simulink model "SF015A_WhlImbRejctn"  (R2013b)
settings: Solver=FixedStepDiscrete  SolverMode=SingleTasking  StartTime=0.0  StopTime=1  FixedStep=0.002  RelTol=1e-3
undefined symbols (not defined in the file): ACTIVBANDMAX_ULS_U32, ADAPVFILMAX_ULS_F32, ADJOUTPMAX_ULS_F32, ARCHGLBPRM_180OVERPI_ULS_F32, ARCHGLBPRM_2MILLISEC_SEC_F32, ARCHGLBPRM_2PI_ULS_F32, ARCHGLBPRM_FLOATZEROTHD_ULS_F32, ARCHGLBPRM_PI_ULS_F32, ARCHGLBPRM_PIOVER180_ULS_F32, ARCHGLBPRM_PIOVER2_ULS_F32, CALMINSPERCOUNT_ULS_F32, Cntr, DURATIONDISABLE_CNT_U16, FILTWHLSPDMAX_MOTRADPERSEC_F32, FRQMIN_ULS_F32, MICROSECTOMILLISEC_ULS_F32, MINSTOMILLISEC_ULS_F32, NINETY_ULS_F32, NODEBSTEP_CNT_U16, NROFDLY_CNT_U08, NtcSts1, NvmGetErrSts1, ONEHALF_ULS_F32, ONEHUNDRED_ULS_F32, ONEOVRTHREE_ULS_F32, ONEOVRTWENTY_ULS_F32, ONETHOUSAND_ULS_F32, PEAKMAX_ULS_F32, PEAKMIN_ULS_F32, PHAADJMAX_ULS_F32, PITIMESSAMPLETIME_ULS_F32, SigQlfr1, STOREDMINSPERCOUNT_ULS_F32, Sts, SysSt1, TWO_ULS_F32, TWOOVRTHREE_ULS_F32, UGRFILMAX_ULS_F32, WhlImbRejctnAdpvFac, WhlImbRejctnAutScaEna, WhlImbRejctnAutScaTar, WhlImbRejctnCurrMgnSlewPerLoop, WhlImbRejctnDcTrendFltRcvryDly, WhlImbRejctnDcTrendFltRcvryNegStep, WhlImbRejctnDcTrendFltRcvryPosStep, WhlImbRejctnDcTrendFltRcvryThd, WhlImbRejctnDcTrendTh2Tq, WhlImbRejctnDcTrendThTq, WhlImbRejctnDcTrendTi2Sec, WhlImbRejctnDcTrendTiSec, WhlImbRejctnEnaSlewPerLoop, WhlImbRejctnFctEna, WhlImbRejctnFltNtc, WhlImbRejctnFrqDiagcAmpThd, WhlImbRejctnFrqDiagcEna, WhlImbRejctnFrqDiagcFltRcvryDly, WhlImbRejctnFrqDiagcFltRcvryNegStep, WhlImbRejctnFrqDiagcFltRcvryPosStep, WhlImbRejctnFrqDiagcFltRcvryThd, WhlImbRejctnFrqDiagcThd ... (+30)
libraries: FixdToFloat x32, simulink x26, NxtrLim x25, Fil x20, NxtrAbslt x9, NxtrMath x7, NxtrMax x6, NxtrMin x4, NxtrNvM x2, FloatToFixd x2, LnrIntrpn x2, NxtrSign x1
(part 1 of 14)
settings Model: Creator=VZBTJX  LastModifiedBy=XZB1DB
settings SolverCC: AutoInsertRateTranBlk=on  InsertRTBMode=Always
settings DataIOCC: LimitDataPoints=off  SaveFormat=Structure  ReturnWorkspaceOutputs=on
settings OptimizationCC: BlockReduction=off  InlineParams=on  ZeroExternalMemoryAtStartup=off  ZeroInternalMemoryAtStartup=off  OptimizeModelRefInitCode=on  LifeSpan=1
settings DebuggingCC: SignalInfNanChecking=error  SignalRangeChecking=warning  UnderspecifiedInitializationDetection=Simplified  SolverPrmCheckMsg=error  InheritedTsInSrcMsg=error  DiscreteInheritContinuousMsg=error  SingleTaskRateTransMsg=error  TasksWithSamePriorityMsg=error  SigSpecEnsureSampleTimeMsg=error  CheckMatrixSingularityMsg=error  ParameterUnderflowMsg=error  ParameterPrecisionLossMsg=error  ParameterTunabilityLossMsg=error  FixptConstUnderflowMsg=warning  FixptConstOverflowMsg=warning  VectorMatrixConversionMsg=error  SignalLabelMismatchMsg=error  UnconnectedInputMsg=error  UnconnectedOutputMsg=error  UnconnectedLineMsg=error  SFcnCompatibilityMsg=error  UniqueDataStoreMsg=warning  BusObjectLabelMismatch=error  RootOutportRequireBusObject=error  AssertControl=DisableAll  ModelReferenceIOMsg=error  ModelReferenceVersionMismatchMessage=warning  ModelReferenceIOMismatchMessage=error  ModelReferenceCSMismatchMessage=warning  ModelReferenceDataLoggingMessage=error  StateNameClashWarn=warning  StrictBusMsg=ErrorOnBusTreatedAsVector  NonBusSignalsTreatedAsBus=error  SFUnexpectedBacktrackingDiag=error  SFInvalidInputDataAccessInChartInitDiag=error  SFNoUnconditionalDefaultTransitionDiag=error  SFTransitionOutsideNaturalParentDiag=error  SFUnconditionalTransitionShadowingDiag=error  SFUndirectedBroadcastEventsDiag=error
settings ModelReferenceCC: ModelReferenceNumInstancesAllowed=Single
settings RTWCC: SystemTargetFile=autosar.tlc  GenCodeOnly=on  TemplateMakefile=ert_default_tmf  Description=AUTOSAR  GenerateReport=on  ProcessScript=autosar_make_rtw_hook  LaunchReport=on
settings CodeAppCC: GenerateComments=off  IgnoreCustomStorageClasses=off  CustomSymbolStrType=$N$R$M  CustomSymbolStrBlkIO=$N$M  SimulinkBlockComments=off
settings STFCustomTargetCC: ParMdlRefBuildCompliant=on  CompOptLevelCompliant=on  IncludeMdlTerminateFcn=off  CombineOutputUpdateFcns=on  SuppressErrorStatus=on  ERTFirstTimeCompliant=on  ERTCustomFileBanners=on  SupportNonFinite=off  SupportComplex=off  SupportContinuousTime=off  SupportNonInlinedSFcns=off  MATLABClassNameForMDSCustomization=Simulink.SoftwareTarget.ERTCustomization  AutosarCompliant=on  GRTInterface=off  SystemTargetFile=autosar.tlc
settings ERTTargetCC: CodeReplacementLibrary=ANSI_C  ConcurrentExecutionCompliant=off  IncludeMdlTerminateFcn=off  SuppressErrorStatus=on  SupportNonFinite=off  SupportComplex=off  ModelStepFunctionPrototypeControlCompliant=off  CPPClassGenCompliant=off  AutosarCompliant=on  InlinedParameterPlacement=NonHierarchical  ERTCustomFileTemplate=example_file_process.tlc  EnableUserReplacementTypes=on

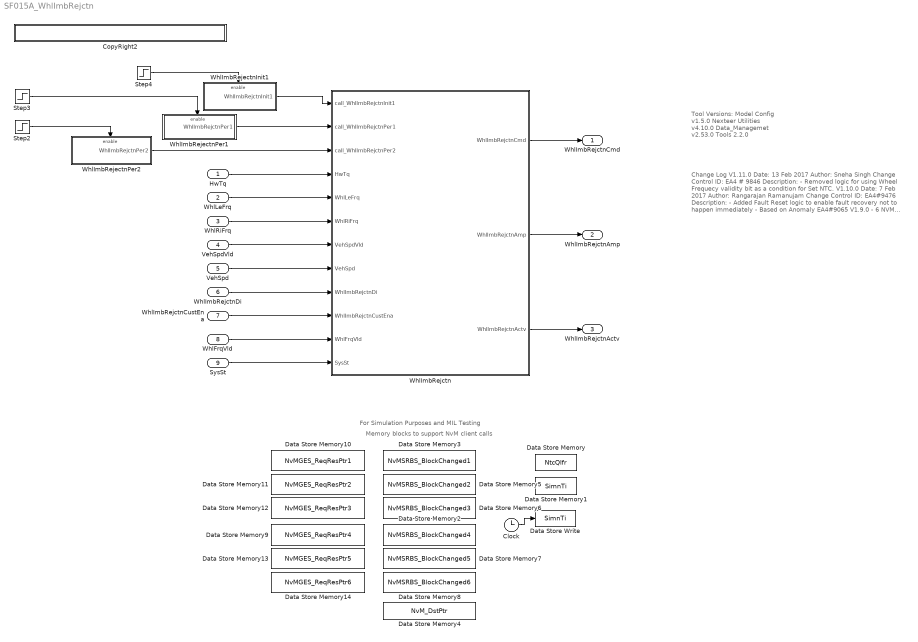
== system SF015A_WhlImbRejctn ==
  note: Tool Versions:
      |
      | Model Config v1.5.0
      | Nexteer Utilities v4.10.0
      | Data_Managemet v2.53.0
      | Tools 2.2.0
  note: Change Log
      |
      | V1.11.0
      | Date: 13 Feb 2017
      | Author: Sneha Singh
      | Change Control ID: EA4 # 9846
      | Description:
      | - Removed logic for using Wheel Frequecy validity bit as a condition for Set NTC.
      |
      | V1.10.0
      | Date: 7 Feb 2017
      | Author: Rangarajan Ramanujam
      | Change Control ID: EA4#9476
      | Description:
      | - Added Fault Reset logic to enable fault recovery not to happen immediately
      | - Based on Anomaly EA4#9065
      |
      |
      | V1.9.0
      | - 6 NVM variables corresponding to Struct 1 NVM block(CmpPeakData).
      | - FRQMIN_ULS_F32 constant added in DD and Model
      | - Input and Output Ports promoted at the top level per Std.
      | - Precision updated  for WhlFreq InRange and WhlFreq InRange 1 Subsystem
      |
      |
      | V1.8.0
      | Date: 28 Nov 2016
      | Author: Rangarajan Ramanujam
      | Change Control ID: EA4#8201
      | Description:
      | - EngMax of DlyIdxLe and DlyIdxRi updated in DD.
      | - Updated the range of PIMs in DD.
      | - Updated IRV properties in DD for 'IniCmpFlt'.
      | - Modified the  '<=' to '>' in PeakLe and PeakRi blocks. The problem exists
      | only in model. No change to code
      | - Updated the EngVal of 'DURATIONDISABLE_CNT_U16' in DD.
      | - Tapped delay implementation has been modified.
      | - Phase Adjust block has been modified.
      | - Updated the block 'Active Rejection Command'.
      | - Modified the Adaptive Filter blocks.
      | - Updated the UGR filter logic.
      | - Deleted few PIMs
      | - Reset WIR block has been updated.
      | - Updated Set NTC blocks without trigger from latest tools
      | - Changed constant value of 'MICROSECTOMILLISEC_ULS_F32' from 0.001 to 0.1
      |
      |
      |
      | V1.7.0
      | Date: 11 October 2016
      | Author: Rangarajan Ramanujam
      | Change Control ID: EA4#7923
      | Description:
      | - PIM Ranges in 'Slow Speed Diagc' update in Data dictionary
      | - Logic update in Data dictionary for not updating PIM when value is at
      | data type max
      | - Add Compensation fault diagnostic to init as per EA3 code
      | - Change NVM checking condition in Init to data type max of u32 instead of
      | u16
      | -The Lowpass filter variable for computing CurrMagLe and CurrMagRi
      | were same and this was resolved with separate Low pass filter state
      | variables for Le and Ri.
      | - Logic for Enabling and disabling WIR updated/changed as per Ea3 code
      |
      | V1.6.0
      | - Minimum Value of LpFil variables checked and changed to prevent
      |  divide by zero issues
      | - Latest tools used to fix LpFil error and prevent LpFilGain being
      | set to zero
      | - Display variable write blocks missing were updated :
      | dWhlImbRejctnLMSqdOutLe and dWhlImbRejctnLMSqdOutRi
      | - Pim Data store memory blocks Diagnostics set to 'none'
      | - Width block used to select first and last elements of an array
      | instead of using 'Arrayname(1)' or 'Arrayname(end)'
      |
      | V1.5.0
      | - 'OR' block replaced with 'Bitwise OR' in the subsystem 'WIR
      | Diagnostics/Set NTC Block'.
      | - Updated the datatype of NTC failure bits to 'uint8' in the 'WIR
      | Diagnostics/Set NTC Block'.
      | - Logic for setting of NTC bit based on WheelFrequencyValid
      | signal has been removed from the subsystem 'WIR Diagnostics'.
      | - Properties of few simulink blocks have been changed to make
      | the model simulatable.
      | - The definition of PIMs of type'Bus:PassFailCntrDiagcRec1' has
      | been updated in the data dictionary.
      |
      |
      | V1.4.0
      | Date: 01 August 2016
      | Author: Rangarajan Ramanujam
      | Change Control: 6681
      | Description:
      | - Rearranging design logic in Wheel speed Correlation check
      |  to remove redundant checks and  match code with model
      |
      | v1.3.0
      | Date: 6 June 2016
      | Author: Sneha Singh
      | Change Control ID: EA4# 5952
      | - NOT block added to the signal WhlImbRejctnDi
      | - Elapsed timer comparison modified from '<=' to '>='.
      | - Changed units of few cals from 'Milliseconds' to 'Mins'.
      | - Logic for conversion of minutes to milliseconds added.
      | - Added a new constant for minutes to milliseconds conversion.
      |
      | V1.2.0
      | Date: 23 Mar 2016
      | Author :Rangarajan Ramanujam
      | Change control :
      | Description:
      | - NVM checks added
      | - Typos fixed in cal names
      | - Design changes in Phase adjust
      | - Initial values updated according to review
      |
      | V1.1.0
      | -Changes corresponding to software review
      |
      | V1.0.0
      | - Initial Release
      | - Based on EA3 Word doc
      | - Level 3 Model
  note: For Simulation Purposes and MIL Testing
  note: Memory blocks to support NvM client calls
  HwTq : Inport
  WhlLeFrq : Inport  Port=2
  WhlRiFrq : Inport  Port=3
  VehSpdVld : Inport  Port=4
  VehSpd : Inport  Port=5
  WhlImbRejctnDi : Inport  Port=6
  WhlImbRejctnCustEna : Inport  Port=7
  WhlFrqVld : Inport  Port=8
  SysSt : Inport  Port=9
  Clock : Clock
  CopyRight2 : Subsystem  Description=|  mask(Copyright Information){none=on}
      | Copyright info block.                                               
      |                                                                     
      | Place copyright information at the top of every subsystem in design.
      mask prompts: none "No parameters"
      mask help: Place copyright information at the top of every subsystem in design.
      mask Display:
      | NxtrConf = 'Nexteer Confidential';
      | 
      | sys = bdroot; %handle for the current model ("system")
      | first = get_param(sys,'Created');
      | first = first(end-3:end);  %year is last four digits
      | 
      | last = get_param(sys,'LastModifiedDate');
      | if isempty(last)
      |     last = datestr(now,'yyyy');
      | else
      |     last = last(end-3:end);
      | end
      | 
      | if strcmp(first,last)
      |     fprintf('%s -- Copyright %s Nexteer',NxtrConf,first)
      | else
      |     fprintf('%s -- %s%s- %s Nexteer',NxtrConf,char(169),first,last)
      | end
  Data Store Memory : DataStoreMemory  DataStoreName=NtcQlfr
  Data Store Memory1 : DataStoreMemory  DataStoreName=SimnTi
  Data Store Memory10 : DataStoreMemory  DataStoreName=NvMGES_ReqResPtr1
  Data Store Memory11 : DataStoreMemory  DataStoreName=NvMGES_ReqResPtr2
  Data Store Memory12 : DataStoreMemory  DataStoreName=NvMGES_ReqResPtr3
  Data Store Memory13 : DataStoreMemory  DataStoreName=NvMGES_ReqResPtr5
  Data Store Memory14 : DataStoreMemory  DataStoreName=NvMGES_ReqResPtr6
  Data Store Memory2 : DataStoreMemory  DataStoreName=NvMSRBS_BlockChanged4
  Data Store Memory3 : DataStoreMemory  DataStoreName=NvMSRBS_BlockChanged1
  Data Store Memory4 : DataStoreMemory  DataStoreName=NvM_DstPtr
  Data Store Memory5 : DataStoreMemory  DataStoreName=NvMSRBS_BlockChanged2
  Data Store Memory6 : DataStoreMemory  DataStoreName=NvMSRBS_BlockChanged3
  Data Store Memory7 : DataStoreMemory  DataStoreName=NvMSRBS_BlockChanged5
  Data Store Memory8 : DataStoreMemory  DataStoreName=NvMSRBS_BlockChanged6
  Data Store Memory9 : DataStoreMemory  DataStoreName=NvMGES_ReqResPtr4
  Data Store Write : DataStoreWrite  DataStoreName=SimnTi
  Step2 : Step  Time=0  SampleTime=0.004
  Step3 : Step  Time=0  SampleTime=0.002
  Step4 : Step  Time=0  Before=1  After=0  SampleTime=0.002
  WhlImbRejctn : Subsystem
  WhlImbRejectnInit1 : Subsystem  RequirementInfo={} %GIDa_18617733_e4ee_4886_bcc3_385a7dcf992d  TreatAsAtomicUnit=on
  WhlImbRejectnPer1 : Subsystem  RequirementInfo={} %GIDa_501e26ae_c5a8_44f7_acd8_34ad9ece32fe  TreatAsAtomicUnit=on
  WhlImbRejectnPer2 : Subsystem  RequirementInfo={} %GIDa_04db69de_43d9_4850_9e5a_188d21d54238  TreatAsAtomicUnit=on
  WhlImbRejctnCmd : Outport
  WhlImbRejctnAmp : Outport  Port=2
  WhlImbRejctnActv : Outport  Port=3
  wires:
  Clock/1 -> Data Store Write/1
  WhlImbRejctn/1(WhlImbRejctnCmd) -> WhlImbRejctnCmd/1
  WhlImbRejctn/2(WhlImbRejctnAmp) -> WhlImbRejctnAmp/1
  WhlImbRejctn/3(WhlImbRejctnActv) -> WhlImbRejctnActv/1
  WhlImbRejectnInit1/1(WhlImbRejctnInit1) -> WhlImbRejctn/1(call_WhlImbRejctnInit1)
  WhlImbRejectnPer1/1(WhlImbRejctnPer1) -> WhlImbRejctn/2(call_WhlImbRejctnPer1)
  WhlImbRejectnPer2/1(WhlImbRejctnPer2) -> WhlImbRejctn/3(call_WhlImbRejctnPer2)
  SysSt/1 -> WhlImbRejctn/12(SysSt)
  HwTq/1 -> WhlImbRejctn/4(HwTq)
  VehSpdVld/1 -> WhlImbRejctn/7(VehSpdVld)
  VehSpd/1 -> WhlImbRejctn/8(VehSpd)
  WhlImbRejctnDi/1 -> WhlImbRejctn/9(WhlImbRejctnDi)
  WhlImbRejctnCustEna/1 -> WhlImbRejctn/10(WhlImbRejctnCustEna)
  WhlFrqVld/1 -> WhlImbRejctn/11(WhlFrqVld)
  Step4/1 -> WhlImbRejectnInit1/Enable
  WhlLeFrq/1 -> WhlImbRejctn/5(WhlLeFrq)
  WhlRiFrq/1 -> WhlImbRejctn/6(WhlRiFrq)
  Step2/1 -> WhlImbRejectnPer2/Enable
  Step3/1 -> WhlImbRejectnPer1/Enable

== system SF015A_WhlImbRejctn/CopyRight2 ==

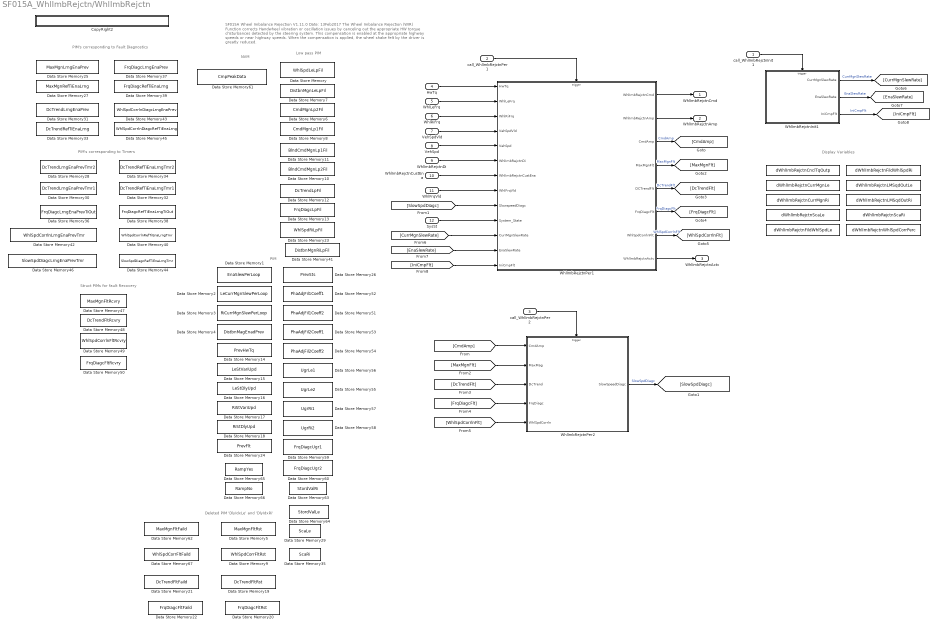
== system SF015A_WhlImbRejctn/WhlImbRejctn ==
  note: Deleted PIM 'DlyIdxLe' and 'DlyIdxRi'
  note: Struct PIMs for fault Recovery
  note: PIM's corresponding to Timers
  note: PIM's corresponding to Fault Diagnostics
  note: NVM
  note: PIM
  note: Display Variables
  note: Low pass PIM
  note: SF015A Wheel Imbalance Rejection
      | V1.11.0 																													    Date: 13Feb2017
      |
      | The Wheel Imbalance Rejection (WIR) Function corrects Handwheel vibration or oscillation issues by canceling out the appropriate HW torque
      | d'isturbances detected by the steering system. This compensation is enabled at the appropriate highway speeds or near highway speeds. When the
      | compensation is applied, the wheel shake felt by the driver is greatly reduced.
  call_WhlImbRejctnInit1 : Inport
  call_WhlImbRejctnPer1 : Inport  Port=2
  call_WhlImbRejctnPer2 : Inport  Port=3
  HwTq : Inport  Port=4
  WhlLeFrq : Inport  Port=5
  WhlRiFrq : Inport  Port=6
  VehSpdVld : Inport  Port=7
  VehSpd : Inport  Port=8
  WhlImbRejctnDi : Inport  Port=9
  WhlImbRejctnCustEna : Inport  Port=10
  WhlFrqVld : Inport  Port=11
  SysSt : Inport  Port=12
  " " : DataStoreMemory  DataStoreName=dWhlImbRejctnCnclTqOutp  StateMustResolveToSignalObject=on
  " " : DataStoreMemory  DataStoreName=dWhlImbRejctnCurrMgnLe  StateMustResolveToSignalObject=on
  " " : DataStoreMemory  DataStoreName=dWhlImbRejctnCurrMgnRi  StateMustResolveToSignalObject=on
  " " : DataStoreMemory  DataStoreName=dWhlImbRejctnFildWhlSpdLe  StateMustResolveToSignalObject=on
  " " : DataStoreMemory  DataStoreName=dWhlImbRejctnFildWhlSpdRi  StateMustResolveToSignalObject=on
  " " : DataStoreMemory  DataStoreName=dWhlImbRejctnLMSqdOutLe  StateMustResolveToSignalObject=on
  " " : DataStoreMemory  DataStoreName=dWhlImbRejctnLMSqdOutRi  StateMustResolveToSignalObject=on
  " " : DataStoreMemory  DataStoreName=dWhlImbRejctnScaLe  StateMustResolveToSignalObject=on
  " " : DataStoreMemory  DataStoreName=dWhlImbRejctnScaRi  StateMustResolveToSignalObject=on
  " " : DataStoreMemory  DataStoreName=dWhlImbRejctnWhlSpdCorrPerc  StateMustResolveToSignalObject=on
  CopyRight2 : Subsystem  Description=|  mask(Copyright Information){none=on}
      | Copyright info block.                                               
      |                                                                     
      | Place copyright information at the top of every subsystem in design.
      mask prompts: none "No parameters"
      mask help: Place copyright information at the top of every subsystem in design.
      mask Display:
      | NxtrConf = 'Nexteer Confidential';
      | 
      | sys = bdroot; %handle for the current model ("system")
      | first = get_param(sys,'Created');
      | first = first(end-3:end);  %year is last four digits
      | 
      | last = get_param(sys,'LastModifiedDate');
      | if isempty(last)
      |     last = datestr(now,'yyyy');
      | else
      |     last = last(end-3:end);
      | end
      | 
      | if strcmp(first,last)
      |     fprintf('%s -- Copyright %s Nexteer',NxtrConf,first)
      | else
      |     fprintf('%s -- %s%s- %s Nexteer',NxtrConf,char(169),first,last)
      | end
  Data Store Memory : DataStoreMemory  DataStoreName=WhlSpdLeLpFil  InitialValue=[]  OutDataTypeStr=Bus: FilLpRec1  StateMustResolveToSignalObject=on
  Data Store Memory1 : DataStoreMemory  DataStoreName=EnaSlewPerLoop  InitialValue=[]  StateMustResolveToSignalObject=on
  Data Store Memory10 : DataStoreMemory  DataStoreName=BlndCmdMgnLp2Fil  InitialValue=[]  OutDataTypeStr=Bus: FilLpRec1  StateMustResolveToSignalObject=on
  Data Store Memory11 : DataStoreMemory  DataStoreName=BlndCmdMgnLp1Fil  InitialValue=[]  OutDataTypeStr=Bus: FilLpRec1  StateMustResolveToSignalObject=on
  Data Store Memory12 : DataStoreMemory  DataStoreName=DcTrendLpFil  InitialValue=[]  OutDataTypeStr=Bus: FilLpRec1  StateMustResolveToSignalObject=on
  Data Store Memory13 : DataStoreMemory  DataStoreName=FrqDiagcLpFil  InitialValue=[]  OutDataTypeStr=Bus: FilLpRec1  StateMustResolveToSignalObject=on
  Data Store Memory14 : DataStoreMemory  DataStoreName=PrevHwTq  InitialValue=[]  StateMustResolveToSignalObject=on
  Data Store Memory15 : DataStoreMemory  DataStoreName=LeStVariUpd  InitialValue=[]  StateMustResolveToSignalObject=on
  Data Store Memory16 : DataStoreMemory  DataStoreName=LeStDlyUpd  InitialValue=[]  StateMustResolveToSignalObject=on
  Data Store Memory17 : DataStoreMemory  DataStoreName=RiStVariUpd  InitialValue=[]  StateMustResolveToSignalObject=on
  Data Store Memory18 : DataStoreMemory  DataStoreName=RiStDlyUpd  InitialValue=[]  StateMustResolveToSignalObject=on
  Data Store Memory19 : DataStoreMemory  DataStoreName=DcTrendFltRst  InitialValue=[]  StateMustResolveToSignalObject=on
  Data Store Memory2 : DataStoreMemory  DataStoreName=LeCurrMgnSlewPerLoop  InitialValue=[]  StateMustResolveToSignalObject=on
  Data Store Memory20 : DataStoreMemory  DataStoreName=FrqDiagcFltRst  InitialValue=[]  StateMustResolveToSignalObject=on
  Data Store Memory21 : DataStoreMemory  DataStoreName=DcTrendFltFaild  InitialValue=[]  StateMustResolveToSignalObject=on
  Data Store Memory22 : DataStoreMemory  DataStoreName=FrqDiagcFltFaild  InitialValue=[]  StateMustResolveToSignalObject=on
  Data Store Memory23 : DataStoreMemory  DataStoreName=WhlSpdRiLpFil  InitialValue=[]  OutDataTypeStr=Bus: FilLpRec1  StateMustResolveToSignalObject=on
  Data Store Memory24 : DataStoreMemory  DataStoreName=PrevFlt  InitialValue=[]  StateMustResolveToSignalObject=on
  Data Store Memory25 : DataStoreMemory  DataStoreName=MaxMgnLrngEnaPrev  InitialValue=[]  StateMustResolveToSignalObject=on
  Data Store Memory26 : DataStoreMemory  DataStoreName=PrevSts  InitialValue=[]  StateMustResolveToSignalObject=on
  Data Store Memory27 : DataStoreMemory  DataStoreName=MaxMgnRefTiEnaLrng  InitialValue=[]  StateMustResolveToSignalObject=on
  Data Store Memory28 : DataStoreMemory  DataStoreName=DcTrendLrngEnaPrevTmr2  InitialValue=[]  StateMustResolveToSignalObject=on
  Data Store Memory29 : DataStoreMemory  DataStoreName=ScaLe  StateMustResolveToSignalObject=on
  Data Store Memory3 : DataStoreMemory  DataStoreName=RiCurrMgnSlewPerLoop  InitialValue=[]  StateMustResolveToSignalObject=on
  Data Store Memory30 : DataStoreMemory  DataStoreName=DcTrendLrngEnaPrevTmr1  InitialValue=[]  StateMustResolveToSignalObject=on
  Data Store Memory31 : DataStoreMemory  DataStoreName=DcTrendLrngEnaPrev  InitialValue=[]  StateMustResolveToSignalObject=on
  Data Store Memory32 : DataStoreMemory  DataStoreName=DcTrendRefTiEnaLrngTmr1  InitialValue=[]  StateMustResolveToSignalObject=on
  Data Store Memory33 : DataStoreMemory  DataStoreName=DcTrendRefTiEnaLrng  InitialValue=[]  StateMustResolveToSignalObject=on
  Data Store Memory34 : DataStoreMemory  DataStoreName=DcTrendRefTiEnaLrngTmr2  InitialValue=[]  StateMustResolveToSignalObject=on
  Data Store Memory35 : DataStoreMemory  DataStoreName=ScaRi  StateMustResolveToSignalObject=on
  Data Store Memory36 : DataStoreMemory  DataStoreName=FrqDiagcLrngEnaPrevTiOut  InitialValue=[]  StateMustResolveToSignalObject=on
  Data Store Memory37 : DataStoreMemory  DataStoreName=FrqDiagcLrngEnaPrev  InitialValue=[]  StateMustResolveToSignalObject=on
  Data Store Memory38 : DataStoreMemory  DataStoreName=FrqDiagcRefTiEnaLrngTiOut  InitialValue=[]  StateMustResolveToSignalObject=on
  Data Store Memory39 : DataStoreMemory  DataStoreName=FrqDiagcRefTiEnaLrng  InitialValue=[]  StateMustResolveToSignalObject=on
  Data Store Memory4 : DataStoreMemory  DataStoreName=DistbnMagEnadPrev  InitialValue=[]  StateMustResolveToSignalObject=on
  Data Store Memory40 : DataStoreMemory  DataStoreName=WhlSpdCorrlnRefTiEnaLrngTmr  InitialValue=[]  StateMustResolveToSignalObject=on
  Data Store Memory41 : DataStoreMemory  DataStoreName=DistbnMgnRiLpFil  InitialValue=[]  OutDataTypeStr=Bus: FilLpRec1  StateMustResolveToSignalObject=on
  Data Store Memory42 : DataStoreMemory  DataStoreName=WhlSpdCorrlnLrngEnaPrevTmr  InitialValue=[]  StateMustResolveToSignalObject=on
  Data Store Memory43 : DataStoreMemory  DataStoreName=WhlSpdCorrlnDiagcLrngEnaPrev  InitialValue=[]  StateMustResolveToSignalObject=on
  Data Store Memory44 : DataStoreMemory  DataStoreName=SlowSpdDiagcRefTiEnaLrngTmr  InitialValue=[]  StateMustResolveToSignalObject=on
  Data Store Memory45 : DataStoreMemory  DataStoreName=WhlSpdCorrlnDiagcRefTiEnaLrng  InitialValue=[]  StateMustResolveToSignalObject=on
  Data Store Memory46 : DataStoreMemory  DataStoreName=SlowSpdDiagcLrngEnaPrevTmr  InitialValue=[]  StateMustResolveToSignalObject=on
  Data Store Memory47 : DataStoreMemory  DataStoreName=MaxMgnFltRcvry  InitialValue=[]  OutDataTypeStr=Bus:PassFailCntrDiagcRec1  StateMustResolveToSignalObject=on
  Data Store Memory48 : DataStoreMemory  DataStoreName=DcTrendFltRcvry  InitialValue=[]  OutDataTypeStr=Bus: PassFailCntrDiagcRec1  StateMustResolveToSignalObject=on
  Data Store Memory49 : DataStoreMemory  DataStoreName=WhlSpdCorrlnFltRcvry  InitialValue=[]  OutDataTypeStr=Bus: PassFailCntrDiagcRec1  StateMustResolveToSignalObject=on
  Data Store Memory5 : DataStoreMemory  DataStoreName=MaxMgnFltRst  InitialValue=[]  StateMustResolveToSignalObject=on
  Data Store Memory50 : DataStoreMemory  DataStoreName=FrqDiagcFltRcvry  InitialValue=[]  OutDataTypeStr=Bus: PassFailCntrDiagcRec1  StateMustResolveToSignalObject=on
  Data Store Memory51 : DataStoreMemory  DataStoreName=PhaAdjFil1Coeff2  InitialValue=[]  StateMustResolveToSignalObject=on
  Data Store Memory52 : DataStoreMemory  DataStoreName=PhaAdjFil1Coeff1  InitialValue=[]  StateMustResolveToSignalObject=on
  Data Store Memory53 : DataStoreMemory  DataStoreName=PhaAdjFil2Coeff1  InitialValue=[]  StateMustResolveToSignalObject=on
  Data Store Memory54 : DataStoreMemory  DataStoreName=PhaAdjFil2Coeff2  InitialValue=[]  StateMustResolveToSignalObject=on
  Data Store Memory55 : DataStoreMemory  DataStoreName=UgrLe2  InitialValue=[]  StateMustResolveToSignalObject=on
  Data Store Memory56 : DataStoreMemory  DataStoreName=UgrLe1  InitialValue=[]  StateMustResolveToSignalObject=on
  Data Store Memory57 : DataStoreMemory  DataStoreName=UgrRi1  InitialValue=[]  StateMustResolveToSignalObject=on
  Data Store Memory58 : DataStoreMemory  DataStoreName=UgrRi2  InitialValue=[]  StateMustResolveToSignalObject=on
  Data Store Memory59 : DataStoreMemory  DataStoreName=FrqDiagcUgr1  InitialValue=[]  StateMustResolveToSignalObject=on
  Data Store Memory6 : DataStoreMemory  DataStoreName=CmdMgnLp2Fil  InitialValue=[]  OutDataTypeStr=Bus: FilLpRec1  StateMustResolveToSignalObject=on
  Data Store Memory60 : DataStoreMemory  DataStoreName=FrqDiagcUgr2  InitialValue=[]  StateMustResolveToSignalObject=on
  Data Store Memory61 : DataStoreMemory  DataStoreName=CmpPeakData  InitialValue=[]  OutDataTypeStr=Bus: WhlImbRejctnCmpPeakRec1  StateMustResolveToSignalObject=on
  Data Store Memory62 : DataStoreMemory  DataStoreName=MaxMgnFltFaild  InitialValue=[]  StateMustResolveToSignalObject=on
  Data Store Memory63 : DataStoreMemory  DataStoreName=StordValRi  InitialValue=[]  StateMustResolveToSignalObject=on
  Data Store Memory64 : DataStoreMemory  DataStoreName=StordValLe  InitialValue=[]  StateMustResolveToSignalObject=on
  Data Store Memory65 : DataStoreMemory  DataStoreName=RampYes  StateMustResolveToSignalObject=on
  Data Store Memory66 : DataStoreMemory  DataStoreName=RampNo  StateMustResolveToSignalObject=on
  Data Store Memory67 : DataStoreMemory  DataStoreName=WhlSpdCorrFltFaild  InitialValue=[]  StateMustResolveToSignalObject=on
  Data Store Memory7 : DataStoreMemory  DataStoreName=DistbnMgnLeLpFil  InitialValue=[]  OutDataTypeStr=Bus: FilLpRec1  StateMustResolveToSignalObject=on
  Data Store Memory8 : DataStoreMemory  DataStoreName=CmdMgnLp1Fil  InitialValue=[]  OutDataTypeStr=Bus: FilLpRec1  StateMustResolveToSignalObject=on
  Data Store Memory9 : DataStoreMemory  DataStoreName=WhlSpdCorrFltRst  InitialValue=[]  StateMustResolveToSignalObject=on
  WhlImbRejctnInit1 : Subsystem
  WhlImbRejctnPer1 : Subsystem
  WhlImbRejctnPer2 : Subsystem  TreatAsAtomicUnit=on
  WhlImbRejctnCmd : Outport
  WhlImbRejctnAmp : Outport  Port=2
  WhlImbRejctnActv : Outport  Port=3
  wires:
  WhlLeFrq/1 -> WhlImbRejctnPer1/2(WhlLeFrq)
  WhlRiFrq/1 -> WhlImbRejctnPer1/3(WhlRiFrq)
  VehSpdVld/1 -> WhlImbRejctnPer1/4(VehSpdVld)
  WhlImbRejctnDi/1 -> WhlImbRejctnPer1/6(WhlImbRejctnDi)
  VehSpd/1 -> WhlImbRejctnPer1/5(VehSpd)
  WhlImbRejctnCustEna/1 -> WhlImbRejctnPer1/7(WhlImbRejctnCustEna)
  HwTq/1 -> WhlImbRejctnPer1/1(HwTq)
  WhlImbRejctnPer1/2(WhlImbRejctnAmp) -> WhlImbRejctnAmp/1
  call_WhlImbRejctnInit1/1 -> WhlImbRejctnInit1/Trigger
  call_WhlImbRejctnPer1/1 -> WhlImbRejctnPer1/Trigger
  WhlFrqVld/1 -> WhlImbRejctnPer1/8(WhlFrqVld)
  call_WhlImbRejctnPer2/1 -> WhlImbRejctnPer2/Trigger
  WhlImbRejctnPer1/3(CmdAmp) -> [CmdAmp]  "CmdAmp"
  [CmdAmp] -> WhlImbRejctnPer2/1(CmdAmp)
  WhlImbRejctnPer2/1("SlowSpeedDiagc ") -> [SlowSpdDiagc]  "SlowSpdDiagc"
  [SlowSpdDiagc] -> WhlImbRejctnPer1/9(SlowspeedDiagc)
  SysSt/1 -> WhlImbRejctnPer1/10(System_State)
  WhlImbRejctnPer1/7(WhlSpdCorrlnFlt) -> [WhlSpdCorrlnFlt]  "WhlSpdCorrlnFlt"
  WhlImbRejctnPer1/6(FrqDiagcFlt) -> [FrqDiagcFlt]  "FrqDiagcFlt"
  WhlImbRejctnPer1/5(DCTrendFlt) -> [DcTrendFlt]  "DcTrendFlt"
  WhlImbRejctnPer1/4(MaxMgnFlt) -> [MaxMgnFlt]  "MaxMgnFlt"
  [MaxMgnFlt] -> WhlImbRejctnPer2/2(MaxMag)
  [DcTrendFlt] -> WhlImbRejctnPer2/3(DcTrend)
  [FrqDiagcFlt] -> WhlImbRejctnPer2/4(FrqDiagc)
  [WhlSpdCorrlnFlt] -> WhlImbRejctnPer2/5(WhlSpdCorrln)
  WhlImbRejctnPer1/8(WhlImbRejctnActv) -> WhlImbRejctnActv/1
  WhlImbRejctnInit1/1(CurrMgnSlewRate) -> [CurrMgnSlewRate]  "CurrMgnSlewRate"
  [CurrMgnSlewRate] -> WhlImbRejctnPer1/11(CurrMgnSlewRate)
  [EnaSlewRate] -> WhlImbRejctnPer1/12(EnaSlewRate)
  WhlImbRejctnInit1/2(EnaSlewRate) -> [EnaSlewRate]  "EnaSlewRate"
  WhlImbRejctnInit1/3(IniCmpFlt) -> [IniCmpFlt]  "IniCmpFlt"
  [IniCmpFlt] -> WhlImbRejctnPer1/13(IniCmpFlt)
  WhlImbRejctnPer1/1(WhlImbRejctnCmd) -> WhlImbRejctnCmd/1

== system SF015A_WhlImbRejctn/WhlImbRejectnInit1 ==
  Enable : EnablePort
  CopyRight2 : Subsystem  Description=|  mask(Copyright Information){none=on}
      | Copyright info block.                                               
      |                                                                     
      | Place copyright information at the top of every subsystem in design.
      mask prompts: none "No parameters"
      mask help: Place copyright information at the top of every subsystem in design.
      mask Display:
      | NxtrConf = 'Nexteer Confidential';
      | 
      | sys = bdroot; %handle for the current model ("system")
      | first = get_param(sys,'Created');
      | first = first(end-3:end);  %year is last four digits
      | 
      | last = get_param(sys,'LastModifiedDate');
      | if isempty(last)
      |     last = datestr(now,'yyyy');
      | else
      |     last = last(end-3:end);
      | end
      | 
      | if strcmp(first,last)
      |     fprintf('%s -- Copyright %s Nexteer',NxtrConf,first)
      | else
      |     fprintf('%s -- %s%s- %s Nexteer',NxtrConf,char(169),first,last)
      | end
  Function-Call Generator : simulink/Ports & Subsystems/Function-Call Generator  sample_time=0.002  numberOfIterations=1
  WhlImbRejctnInit1 : Outport
  wires:
  Function-Call Generator/1 -> WhlImbRejctnInit1/1

== system SF015A_WhlImbRejctn/WhlImbRejectnPer1 ==
  Enable : EnablePort
  CopyRight2 : Subsystem  Description=|  mask(Copyright Information){none=on}
      | Copyright info block.                                               
      |                                                                     
      | Place copyright information at the top of every subsystem in design.
      mask prompts: none "No parameters"
      mask help: Place copyright information at the top of every subsystem in design.
      mask Display:
      | NxtrConf = 'Nexteer Confidential';
      | 
      | sys = bdroot; %handle for the current model ("system")
      | first = get_param(sys,'Created');
      | first = first(end-3:end);  %year is last four digits
      | 
      | last = get_param(sys,'LastModifiedDate');
      | if isempty(last)
      |     last = datestr(now,'yyyy');
      | else
      |     last = last(end-3:end);
      | end
      | 
      | if strcmp(first,last)
      |     fprintf('%s -- Copyright %s Nexteer',NxtrConf,first)
      | else
      |     fprintf('%s -- %s%s- %s Nexteer',NxtrConf,char(169),first,last)
      | end
  Function-Call Generator : simulink/Ports & Subsystems/Function-Call Generator  sample_time=0.002  numberOfIterations=1
  WhlImbRejctnPer1 : Outport
  wires:
  Function-Call Generator/1 -> WhlImbRejctnPer1/1

== system SF015A_WhlImbRejctn/WhlImbRejectnPer2 ==
  Enable : EnablePort
  CopyRight2 : Subsystem  Description=|  mask(Copyright Information){none=on}
      | Copyright info block.                                               
      |                                                                     
      | Place copyright information at the top of every subsystem in design.
      mask prompts: none "No parameters"
      mask help: Place copyright information at the top of every subsystem in design.
      mask Display:
      | NxtrConf = 'Nexteer Confidential';
      | 
      | sys = bdroot; %handle for the current model ("system")
      | first = get_param(sys,'Created');
      | first = first(end-3:end);  %year is last four digits
      | 
      | last = get_param(sys,'LastModifiedDate');
      | if isempty(last)
      |     last = datestr(now,'yyyy');
      | else
      |     last = last(end-3:end);
      | end
      | 
      | if strcmp(first,last)
      |     fprintf('%s -- Copyright %s Nexteer',NxtrConf,first)
      | else
      |     fprintf('%s -- %s%s- %s Nexteer',NxtrConf,char(169),first,last)
      | end
  Function-Call Generator : simulink/Ports & Subsystems/Function-Call Generator  sample_time=0.004  numberOfIterations=1
  WhlImbRejctnPer2 : Outport
  wires:
  Function-Call Generator/1 -> WhlImbRejctnPer2/1

== system SF015A_WhlImbRejctn/WhlImbRejctn/CopyRight2 ==

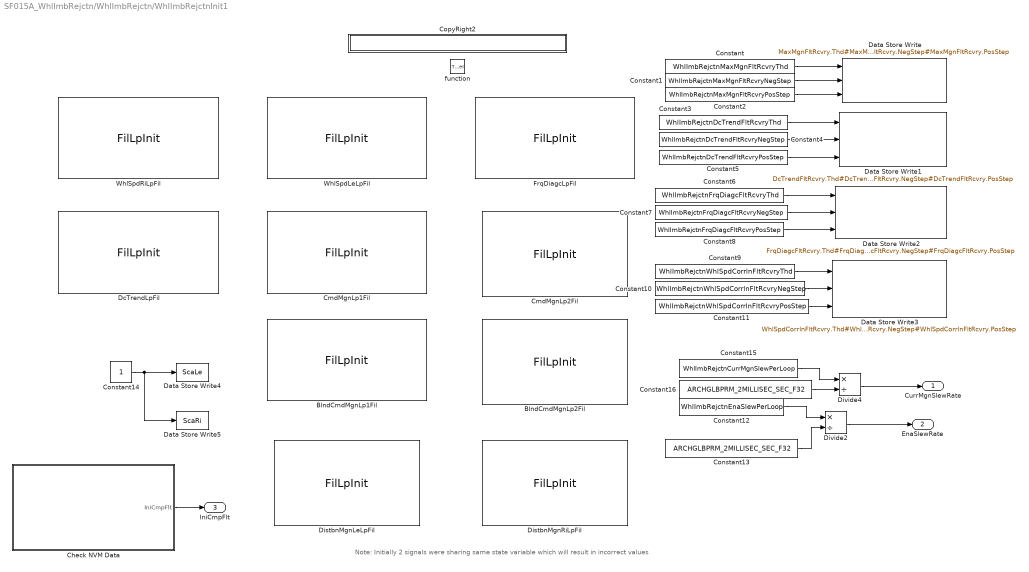
== system SF015A_WhlImbRejctn/WhlImbRejctn/WhlImbRejctnInit1 ==
  note: Note: Initially 2 signals were sharing same state variable which will result in incorrect values
  function : TriggerPort  TriggerType=function-call
  BlndCmdMgnLp1Fil : Fil/FilLpInit  Ic=0  Ts=ARCHGLBPRM_2MILLISEC_SEC_F32  Freq=WhlImbRejctnBlndCmdMgnLp1FilFrq  StVar=BlndCmdMgnLp1Fil
  BlndCmdMgnLp2Fil : Fil/FilLpInit  Ic=0  Ts=ARCHGLBPRM_2MILLISEC_SEC_F32  Freq=WhlImbRejctnBlndCmdMgnLp2FilFrq  StVar=BlndCmdMgnLp2Fil
  Check NVM Data : Subsystem
  CmdMgnLp1Fil : Fil/FilLpInit  Ic=0  Ts=ARCHGLBPRM_2MILLISEC_SEC_F32  Freq=WhlImbRejctnCmdMgnLp1FilFrq  StVar=CmdMgnLp1Fil
  CmdMgnLp2Fil : Fil/FilLpInit  Ic=0  Ts=ARCHGLBPRM_2MILLISEC_SEC_F32  Freq=WhlImbRejctnCmdMgnLp2FilFrq  StVar=CmdMgnLp2Fil
  Constant : Constant  Value=WhlImbRejctnMaxMgnFltRcvryThd
  Constant1 : Constant  Value=WhlImbRejctnMaxMgnFltRcvryNegStep
  Constant10 : Constant  Value=WhlImbRejctnWhlSpdCorrlnFltRcvryNegStep
  Constant11 : Constant  Value=WhlImbRejctnWhlSpdCorrlnFltRcvryPosStep
  Constant12 : Constant  Value=WhlImbRejctnEnaSlewPerLoop
  Constant13 : Constant  Value=ARCHGLBPRM_2MILLISEC_SEC_F32
  Constant14 : Constant  OutDataTypeStr=single
  Constant15 : Constant  Value=WhlImbRejctnCurrMgnSlewPerLoop
  Constant16 : Constant  Value=ARCHGLBPRM_2MILLISEC_SEC_F32
  Constant2 : Constant  Value=WhlImbRejctnMaxMgnFltRcvryPosStep  OutDataTypeStr=single
  Constant3 : Constant  Value=WhlImbRejctnDcTrendFltRcvryThd
  Constant4 : Constant  Value=WhlImbRejctnDcTrendFltRcvryNegStep
  Constant5 : Constant  Value=WhlImbRejctnDcTrendFltRcvryPosStep
  Constant6 : Constant  Value=WhlImbRejctnFrqDiagcFltRcvryThd
  Constant7 : Constant  Value=WhlImbRejctnFrqDiagcFltRcvryNegStep
  Constant8 : Constant  Value=WhlImbRejctnFrqDiagcFltRcvryPosStep
  Constant9 : Constant  Value=WhlImbRejctnWhlSpdCorrlnFltRcvryThd
  CopyRight2 : Subsystem  Description=|  mask(Copyright Information){none=on}
      | Copyright info block.                                               
      |                                                                     
      | Place copyright information at the top of every subsystem in design.
      mask prompts: none "No parameters"
      mask help: Place copyright information at the top of every subsystem in design.
      mask Display:
      | NxtrConf = 'Nexteer Confidential';
      | 
      | sys = bdroot; %handle for the current model ("system")
      | first = get_param(sys,'Created');
      | if(isempty(first))
      |     first = datestr(now,'yyyy');
      | else
      |     first = first(end-3:end);  %year is last four digits
      | end
      | 
      | last = get_param(sys,'LastModifiedDate');
      | if isempty(last)
      |     last = datestr(now,'yyyy');
      | else
      |     last = last(end-3:end);
      | end
      | 
      | if strcmp(first,last)
      |     fprintf('%s -- Copyright %s Nexteer',NxtrConf,first)
      | else
      |     fprintf('%s -- %s%s- %s Nexteer',NxtrConf,char(169),first,last)
      | end
  Data Store Write : DataStoreWrite  DataStoreName=MaxMgnFltRcvry  DataStoreElements=MaxMgnFltRcvry.Thd#MaxMgnFltRcvry.NegStep#MaxMgnFltRcvry.PosStep
  Data Store Write1 : DataStoreWrite  DataStoreName=DcTrendFltRcvry  DataStoreElements=DcTrendFltRcvry.Thd#DcTrendFltRcvry.NegStep#DcTrendFltRcvry.PosStep
  Data Store Write2 : DataStoreWrite  DataStoreName=FrqDiagcFltRcvry  DataStoreElements=FrqDiagcFltRcvry.Thd#FrqDiagcFltRcvry.NegStep#FrqDiagcFltRcvry.PosStep
  Data Store Write3 : DataStoreWrite  DataStoreName=WhlSpdCorrlnFltRcvry  DataStoreElements=WhlSpdCorrlnFltRcvry.Thd#WhlSpdCorrlnFltRcvry.NegStep#WhlSpdCorrlnFltRcvry.PosStep
  Data Store Write4 : DataStoreWrite  DataStoreName=ScaLe
      settings: AttributesFormatString=%<Priority>
  Data Store Write5 : DataStoreWrite  DataStoreName=ScaRi
      settings: AttributesFormatString=%<Priority>
  DcTrendLpFil : Fil/FilLpInit  Ic=0  Ts=ARCHGLBPRM_2MILLISEC_SEC_F32  Freq=WhlImbRejctnDcTrendLpFil  StVar=DcTrendLpFil
  DistbnMgnLeLpFil : Fil/FilLpInit  Ic=0  Ts=ARCHGLBPRM_2MILLISEC_SEC_F32  Freq=WhlImbRejctnDistbnMgnLpFil  StVar=DistbnMgnLeLpFil
  DistbnMgnRiLpFil : Fil/FilLpInit  Ic=0  Ts=ARCHGLBPRM_2MILLISEC_SEC_F32  Freq=WhlImbRejctnDistbnMgnLpFil  StVar=DistbnMgnRiLpFil
  Divide2 : Product  Inputs=*/
  Divide4 : Product  Inputs=*/
  FrqDiagcLpFil : Fil/FilLpInit  Ic=0  Ts=ARCHGLBPRM_2MILLISEC_SEC_F32  Freq=WhlImbRejctnFrqDiagcLpFil  StVar=FrqDiagcLpFil
  WhlSpdLeLpFil : Fil/FilLpInit  Ic=0  Ts=ARCHGLBPRM_2MILLISEC_SEC_F32  Freq=WhlImbRejctnWhlSpdLpFil  StVar=WhlSpdLeLpFil
  WhlSpdRiLpFil : Fil/FilLpInit  Ic=0  Ts=ARCHGLBPRM_2MILLISEC_SEC_F32  Freq=WhlImbRejctnWhlSpdLpFil  StVar=WhlSpdRiLpFil
  CurrMgnSlewRate : Outport
  EnaSlewRate : Outport  Port=2
  IniCmpFlt : Outport  Port=3
  wires:
  Constant15/1 -> Divide4/1
  Constant16/1 -> Divide4/2
  Divide4/1 -> CurrMgnSlewRate/1
  Constant12/1 -> Divide2/1
  Constant13/1 -> Divide2/2
  Divide2/1 -> EnaSlewRate/1
  Constant14/1 -> Data Store Write5/1, Data Store Write4/1
  Constant/1 -> Data Store Write/1
  Constant1/1 -> Data Store Write/2
  Constant2/1 -> Data Store Write/3
  Constant5/1 -> Data Store Write1/3
  Constant4/1 -> Data Store Write1/2
  Constant3/1 -> Data Store Write1/1
  Constant7/1 -> Data Store Write2/2
  Constant8/1 -> Data Store Write2/3
  Constant6/1 -> Data Store Write2/1
  Constant11/1 -> Data Store Write3/3
  Constant10/1 -> Data Store Write3/2
  Constant9/1 -> Data Store Write3/1
  Check NVM Data/1(IniCmpFlt) -> IniCmpFlt/1

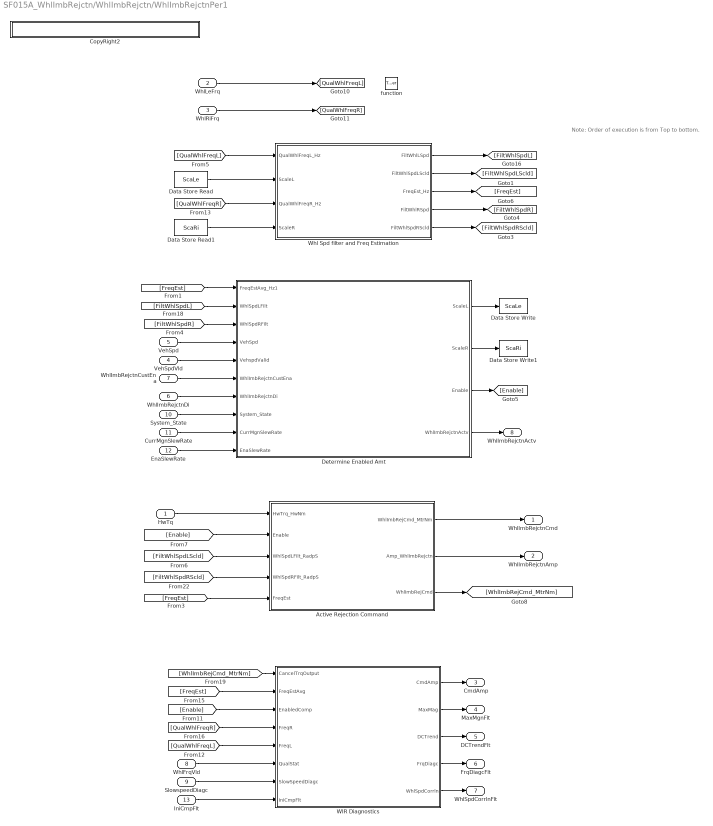
== system SF015A_WhlImbRejctn/WhlImbRejctn/WhlImbRejctnPer1 ==
  note: Note: Order of execution is from Top to bottom.
  HwTq : Inport
  WhlLeFrq : Inport  Port=2
  WhlRiFrq : Inport  Port=3
  VehSpdVld : Inport  Port=4
  VehSpd : Inport  Port=5
  WhlImbRejctnDi : Inport  Port=6
  WhlImbRejctnCustEna : Inport  Port=7
  WhlFrqVld : Inport  Port=8
  SlowspeedDiagc : Inport  Port=9
  System_State : Inport  Port=10
  CurrMgnSlewRate : Inport  Port=11
  EnaSlewRate : Inport  Port=12
  IniCmpFlt : Inport  Port=13
  function : TriggerPort  TriggerType=function-call
  "Active Rejection Command " : Subsystem
  CopyRight2 : Subsystem  Description=|  mask(Copyright Information){none=on}
      | Copyright info block.                                               
      |                                                                     
      | Place copyright information at the top of every subsystem in design.
      mask prompts: none "No parameters"
      mask help: Place copyright information at the top of every subsystem in design.
      mask Display:
      | NxtrConf = 'Nexteer Confidential';
      | 
      | sys = bdroot; %handle for the current model ("system")
      | first = get_param(sys,'Created');
      | first = first(end-3:end);  %year is last four digits
      | 
      | last = get_param(sys,'LastModifiedDate');
      | if isempty(last)
      |     last = datestr(now,'yyyy');
      | else
      |     last = last(end-3:end);
      | end
      | 
      | if strcmp(first,last)
      |     fprintf('%s -- Copyright %s Nexteer',NxtrConf,first)
      | else
      |     fprintf('%s -- %s%s- %s Nexteer',NxtrConf,char(169),first,last)
      | end
  Data Store Read : DataStoreRead  Priority=1  DataStoreName=ScaLe
      settings: AttributesFormatString=%<Priority>
  Data Store Read1 : DataStoreRead  Priority=1  DataStoreName=ScaRi
      settings: AttributesFormatString=%<Priority>
  Data Store Write : DataStoreWrite  Priority=2  DataStoreName=ScaLe
      settings: AttributesFormatString=%<Priority>
  Data Store Write1 : DataStoreWrite  Priority=2  DataStoreName=ScaRi
      settings: AttributesFormatString=%<Priority>
  Determine Enabled Amt : Subsystem
  WIR Diagnostics : Subsystem
  Whl Spd filter and Freq Estimation : Subsystem
  WhlImbRejctnCmd : Outport
  WhlImbRejctnAmp : Outport  Port=2
  CmdAmp : Outport  Port=3
  MaxMgnFlt : Outport  Port=4
  DCTrendFlt : Outport  Port=5
  FrqDiagcFlt : Outport  Port=6
  WhlSpdCorrlnFlt : Outport  Port=7
  WhlImbRejctnActv : Outport  Port=8
  wires:
  Determine Enabled Amt/3(Enable) -> [Enable]
  WhlLeFrq/1 -> [QualWhlFreqL]
  [FiltWhlSpdRScld] -> "Active Rejection Command "/4(WhlSpdRFilt_RadpS)
  "Active Rejection Command "/1(WhlImbRejCmd_MtrNm) -> WhlImbRejctnCmd/1
  Determine Enabled Amt/2(ScaleR) -> Data Store Write1/1
  Whl Spd filter and Freq Estimation/1(FiltWhlLSpd) -> [FiltWhlSpdL]
  Whl Spd filter and Freq Estimation/4(FiltWhlRSpd) -> [FiltWhlSpdR]
  Data Store Read1/1 -> Whl Spd filter and Freq Estimation/4(ScaleR)
  HwTq/1 -> "Active Rejection Command "/1(HwTrq_HwNm)
  Whl Spd filter and Freq Estimation/5(FiltWhlSpdRScld) -> [FiltWhlSpdRScld]
  Data Store Read/1 -> Whl Spd filter and Freq Estimation/2(ScaleL)
  [FiltWhlSpdR] -> Determine Enabled Amt/3(WhlSpdRFilt)
  Determine Enabled Amt/1(ScaleL) -> Data Store Write/1
  VehSpd/1 -> Determine Enabled Amt/4(VehSpd)
  [FiltWhlSpdL] -> Determine Enabled Amt/2(WhlSpdLFilt)
  [FiltWhlSpdLScld] -> "Active Rejection Command "/3(WhlSpdLFilt_RadpS)
  [Enable] -> "Active Rejection Command "/2(Enable)
  Whl Spd filter and Freq Estimation/2(FiltWhlSpdLScld) -> [FiltWhlSpdLScld]
  "Active Rejection Command "/2(Amp_WhlImbRejctn) -> WhlImbRejctnAmp/1
  WhlRiFrq/1 -> [QualWhlFreqR]
  VehSpdVld/1 -> Determine Enabled Amt/5(VehspdValid)
  WhlImbRejctnCustEna/1 -> Determine Enabled Amt/6(WhlImbRejctnCustEna)
  WhlImbRejctnDi/1 -> Determine Enabled Amt/7(WhlImbRejctnDi)
  Whl Spd filter and Freq Estimation/3(FreqEst_Hz) -> [FreqEst]
  [FreqEst] -> Determine Enabled Amt/1(FreqEstAvg_Hz1)
  [FreqEst] -> "Active Rejection Command "/5(FreqEst)
  [WhlImbRejCmd_MtrNm] -> WIR Diagnostics/1(CancelTrqOutput)
  [FreqEst] -> WIR Diagnostics/2(FreqEstAvg)
  [Enable] -> WIR Diagnostics/3(EnabledComp)
  [QualWhlFreqR] -> WIR Diagnostics/4(FreqR)
  [QualWhlFreqL] -> WIR Diagnostics/5(FreqL)
  WhlFrqVld/1 -> WIR Diagnostics/6(QualStat)
  WIR Diagnostics/1(CmdAmp) -> CmdAmp/1
  SlowspeedDiagc/1 -> WIR Diagnostics/7("SlowSpeedDiagc ")
  System_State/1 -> Determine Enabled Amt/8(System_State)
  WIR Diagnostics/2(MaxMag) -> MaxMgnFlt/1
  WIR Diagnostics/3(DCTrend) -> DCTrendFlt/1
  WIR Diagnostics/4(FrqDiagc) -> FrqDiagcFlt/1
  WIR Diagnostics/5(WhlSpdCorrln) -> WhlSpdCorrlnFlt/1
  [QualWhlFreqL] -> Whl Spd filter and Freq Estimation/1(QualWhlFreqL_Hz)
  [QualWhlFreqR] -> Whl Spd filter and Freq Estimation/3(QualWhlFreqR_Hz)
  Determine Enabled Amt/4(WhlImbRejctnActv) -> WhlImbRejctnActv/1
  CurrMgnSlewRate/1 -> Determine Enabled Amt/9(CurrMgnSlewRate)
  EnaSlewRate/1 -> Determine Enabled Amt/10(EnaSlewRate)
  IniCmpFlt/1 -> WIR Diagnostics/8(IniCmpFlt)
  "Active Rejection Command "/3(WhlImbRejCmd) -> [WhlImbRejCmd_MtrNm]

== system SF015A_WhlImbRejctn/WhlImbRejctn/WhlImbRejctnPer2 ==
  CmdAmp : Inport
  MaxMag : Inport  Port=2
  DcTrend : Inport  Port=3
  FrqDiagc : Inport  Port=4
  WhlSpdCorrln : Inport  Port=5
  function : TriggerPort  TriggerType=function-call
  Constant12 : Constant  Value=WhlImbRejctnWhlSpdCorrlnFltRcvryDly
  Constant5 : Constant  Value=WhlImbRejctnMaxMgnFltRcvryDly
  Constant6 : Constant  Value=WhlImbRejctnDcTrendFltRcvryDly
  Constant9 : Constant  Value=WhlImbRejctnFrqDiagcFltRcvryDly
  CopyRight2 : Subsystem  Description=|  mask(Copyright Information){none=on}
      | Copyright info block.                                               
      |                                                                     
      | Place copyright information at the top of every subsystem in design.
      mask prompts: none "No parameters"
      mask help: Place copyright information at the top of every subsystem in design.
      mask Display:
      | NxtrConf = 'Nexteer Confidential';
      | 
      | sys = bdroot; %handle for the current model ("system")
      | first = get_param(sys,'Created');
      | first = first(end-3:end);  %year is last four digits
      | 
      | last = get_param(sys,'LastModifiedDate');
      | if isempty(last)
      |     last = datestr(now,'yyyy');
      | else
      |     last = last(end-3:end);
      | end
      | 
      | if strcmp(first,last)
      |     fprintf('%s -- Copyright %s Nexteer',NxtrConf,first)
      | else
      |     fprintf('%s -- %s%s- %s Nexteer',NxtrConf,char(169),first,last)
      | end
  Flt Recovery- DC Trend : Subsystem
  Flt Recovery- Freq Diag : Subsystem
  Flt Recovery- Max Mag : Subsystem
  Flt Recovery- WhlSpdCorr Diag : Subsystem
  WIR Low Speed Diagnostics : Subsystem
  "SlowSpeedDiagc " : Outport
  wires:
  Constant5/1 -> Flt Recovery- Max Mag/2(FltRecDly)
  MaxMag/1 -> Flt Recovery- Max Mag/1(FltStatIn)
  Constant6/1 -> Flt Recovery- DC Trend/2(FltRecDly)
  Constant9/1 -> Flt Recovery- Freq Diag/2(FltRecDly)
  Constant12/1 -> Flt Recovery- WhlSpdCorr Diag/2(FltRecDly)
  DcTrend/1 -> Flt Recovery- DC Trend/1(FltStatIn)
  FrqDiagc/1 -> Flt Recovery- Freq Diag/1(FltStatIn)
  WhlSpdCorrln/1 -> Flt Recovery- WhlSpdCorr Diag/1(FltStatIn)
  CmdAmp/1 -> WIR Low Speed Diagnostics/1(CmdAmp)
  WIR Low Speed Diagnostics/1(WIRFltStatus_SlowSpeed) -> "SlowSpeedDiagc "/1

== system SF015A_WhlImbRejctn/WhlImbRejectnInit1/CopyRight2 ==

== system SF015A_WhlImbRejctn/WhlImbRejectnPer1/CopyRight2 ==

== system SF015A_WhlImbRejctn/WhlImbRejectnPer2/CopyRight2 ==
